simulink model "gif_model"  (R2013a)
settings: Solver=VariableStepDiscrete  StartTime=0.0  StopTime=t_f  RelTol=1e-3
values from neighbouring files (symbols this model uses):
  dt = 1    [test.m]
undefined symbols (not defined in the file or in its folder): filename_main, filename_target, initial_epoch, VERBOSE
libraries: commutil2 x2, dspswit3 x1
settings Model: Creator=Nathan  LastModifiedBy=Adam
settings DataIOCC: LimitDataPoints=off

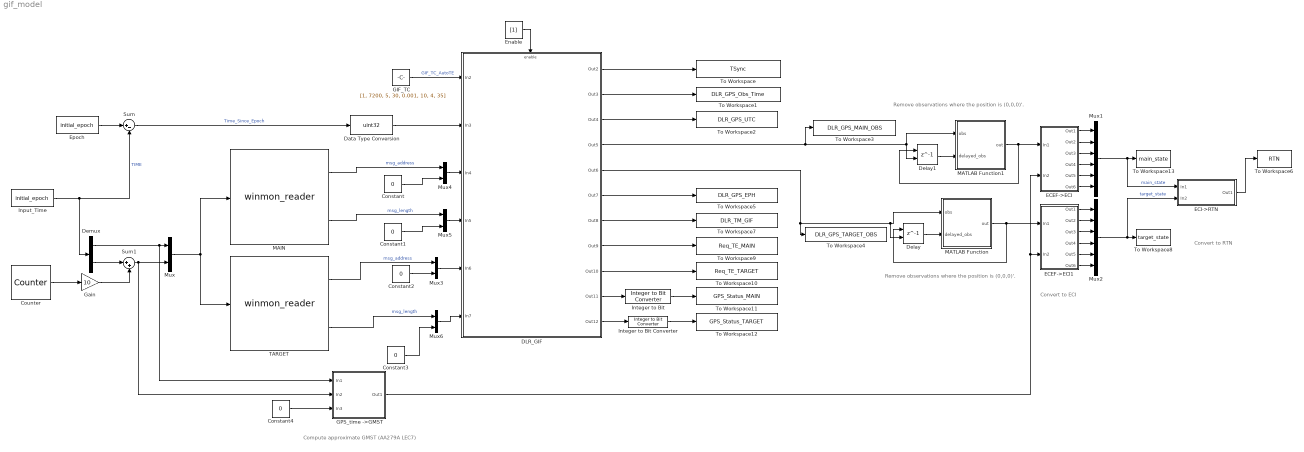
== system gif_model ==
  note: Remove observations where the position is (0,0,0)'.
  note: Convert to RTN
  note: Convert to ECI
  note: Compute approximate GMST
      | (AA279A LEC7)
  note: Remove observations where the position is (0,0,0)'.
  Constant{,1..3} (4 alike) : Constant  Value=0  OutDataTypeStr=uint32
  Constant4 : Constant  Value=0
  Counter : dspswit3/Counter  Direction=Up  CountEvent=Free running  CounterSize=User defined  MaxCount=t_f  InitialCount=0  Output=Count  HitValue=32  ResetInput=off  SamplesPerFrame=1  Ts=10  CntDtype=double  HitDtype=Logical
  DLR_GIF : Subsystem
      mask Display:
      | port_label('input',1,'TC_DLR_GIF')
      | port_label('input',2,'GPS_TIME')
      | port_label('input',3,'GPS_msg_adr_MAIN')
      | port_label('input',4,'GPS_msg_len_MAIN')
      | port_label('input',5,'GPS_msg_adr_TARGET')
      | port_label('input',6,'GPS_msg_len_TARGET')
      | 
      | port_label('output',1,'TSync')
      | port_label('output',2,'DLR_GPS_Obs_Time')
      | port_label('output',3,'DLR_GPS_UTC')
      | port_label('output',4,'DLR_GPS_MAIN_OBS')
      | port_label('output',5,'DLR_GPS_TARGET_OBS')
      | port_label('output',6,'DLR_GPS_EPH')
      | port_label('output',7,'DLR_TM_GIF')
      | port_label('output',8,'Req TE_MAIN')
      | port_label('output',9,'Req TE_TARGET')
      | port_label('output',10,'GPS_Status_MAIN')
      | port_label('output',11,'GPS_Status_TARGET')
  Data Type Conversion : DataTypeConversion  OutDataTypeStr=uint32
  Delay : Delay  DelayLength=1  InitialConditionSource=Input port
      settings: InputPortMap=u0,p4
  Delay1 : Delay  DelayLength=1  InitialConditionSource=Input port
      settings: InputPortMap=u0,p4
  Demux : Demux  Outputs=2
  ECEF->ECI : Subsystem
  ECEF->ECI1 : Subsystem
  ECI->RTN : Subsystem
  Enable : Constant  Value=[1]  OutDataTypeStr=double
  Epoch : Constant  Value=initial_epoch  OutDataTypeStr=double
  "GIF_TC " : Constant  Value=[1, 7200, 5, 30, 0.001, 10, 4, 35]  OutDataTypeStr=double
  GPS_time ->GMST : Subsystem
  Gain : Gain  Gain=10
  "Input_Time " : Constant  Value=initial_epoch  OutDataTypeStr=double
  Integer to Bit : commutil2/Integer to Bit Converter  nbits=7  signedInputValues=Unsigned  bitOrder=MSB first  outDtype=Inherit via internal rule
  Integer to Bit Converter : commutil2/Integer to Bit Converter  nbits=7  signedInputValues=Unsigned  bitOrder=MSB first  outDtype=Inherit via internal rule
  "MAIN " : S-Function  FunctionName=winmon_reader  Parameters=filename_main,dt,VERBOSE  EnableBusSupport=off
  MATLAB Function : MATLAB Function  TreatAsAtomicUnit=on
  MATLAB Function1 : MATLAB Function  TreatAsAtomicUnit=on
  Mux{,3..6} (5 alike) : Mux  Inputs=2
  Mux1 : Mux  Inputs=6
  Mux2 : Mux  Inputs=6
  Sum : Sum  Inputs=|+-
  Sum1 : Sum  Inputs=|++
  TARGET : S-Function  FunctionName=winmon_reader  Parameters=filename_target,dt,VERBOSE  EnableBusSupport=off
  To Workspace : ToWorkspace  VariableName=TSync  SampleTime=-1
  To Workspace1 : ToWorkspace  VariableName=DLR_GPS_Obs_Time  SampleTime=-1
  To Workspace10 : ToWorkspace  VariableName=Req_TE_TARGET  SampleTime=-1
  To Workspace11 : ToWorkspace  VariableName=GPS_Status_MAIN  SampleTime=-1
  To Workspace12 : ToWorkspace  VariableName=GPS_Status_TARGET  SampleTime=-1
  To Workspace13 : ToWorkspace  VariableName=main_state  SampleTime=-1
  To Workspace2 : ToWorkspace  VariableName=DLR_GPS_UTC  SampleTime=-1
  To Workspace3 : ToWorkspace  VariableName=DLR_GPS_MAIN_OBS  SampleTime=-1
  To Workspace4 : ToWorkspace  VariableName=DLR_GPS_TARGET_OBS  SampleTime=-1
  To Workspace5 : ToWorkspace  VariableName=DLR_GPS_EPH  SampleTime=-1
  To Workspace6 : ToWorkspace  VariableName=RTN  SampleTime=-1
  To Workspace7 : ToWorkspace  VariableName=DLR_TM_GIF  SampleTime=-1
  To Workspace8 : ToWorkspace  VariableName=target_state  SampleTime=-1
  To Workspace9 : ToWorkspace  VariableName=Req_TE_MAIN  SampleTime=-1
  wires:
  "Input_Time "/1 -> Demux/1, Sum/2  "TIME"
  Epoch/1 -> Sum/1
  Sum/1 -> Data Type Conversion/1  "Time_Since_Epoch"
  "GIF_TC "/1 -> DLR_GIF/1(In2)  "GIF_TC_AutoTE"
  Enable/1 -> DLR_GIF/Enable
  "MAIN "/1 -> Mux4/1  "msg_address"
  Counter/1 -> Gain/1
  Gain/1 -> Sum1/2
  Demux/2 -> Sum1/1
  Demux/1 -> GPS_time ->GMST/1(In1), Mux/1
  Mux/1 -> "MAIN "/1, TARGET/1
  DLR_GIF/7(Out8) -> To Workspace7/1
  Constant/1 -> Mux4/2
  "MAIN "/2 -> Mux5/1  "msg_length"
  Constant1/1 -> Mux5/2
  TARGET/1 -> Mux3/1  "msg_address"
  Constant2/1 -> Mux3/2
  TARGET/2 -> Mux6/1  "msg_length"
  Constant3/1 -> Mux6/2
  Data Type Conversion/1 -> DLR_GIF/2(In3)
  DLR_GIF/1(Out2) -> To Workspace/1
  DLR_GIF/2(Out3) -> To Workspace1/1
  DLR_GIF/3(Out4) -> To Workspace2/1
  DLR_GIF/4(Out5) -> Delay1/2, MATLAB Function1/1(obs), To Workspace3/1
  DLR_GIF/5(Out6) -> Delay/2, MATLAB Function/1(obs), To Workspace4/1
  DLR_GIF/6(Out7) -> To Workspace5/1
  DLR_GIF/8(Out9) -> To Workspace9/1
  DLR_GIF/9(Out10) -> To Workspace10/1
  ECEF->ECI/1(Out1) -> Mux1/1
  ECEF->ECI/6(Out6) -> Mux1/6
  ECEF->ECI/4(Out4) -> Mux1/4
  ECEF->ECI/3(Out3) -> Mux1/3
  ECEF->ECI/2(Out2) -> Mux1/2
  ECEF->ECI/5(Out5) -> Mux1/5
  Mux1/1 -> ECI->RTN/1(In1), To Workspace13/1  "main_state"
  Sum1/1 -> GPS_time ->GMST/2(In2), Mux/2
  Mux2/1 -> ECI->RTN/2(In2), To Workspace8/1  "target_state"
  ECEF->ECI1/1(Out1) -> Mux2/1
  ECEF->ECI1/3(Out3) -> Mux2/3
  ECEF->ECI1/4(Out4) -> Mux2/4
  ECEF->ECI1/5(Out5) -> Mux2/5
  ECEF->ECI1/2(Out2) -> Mux2/2
  ECEF->ECI1/6(Out6) -> Mux2/6
  Mux6/1 -> DLR_GIF/6(In7)
  Mux4/1 -> DLR_GIF/3(In4)
  Mux5/1 -> DLR_GIF/4(In5)
  Mux3/1 -> DLR_GIF/5(In6)
  ECI->RTN/1(Out1) -> To Workspace6/1
  DLR_GIF/10(Out11) -> Integer to Bit/1
  Integer to Bit/1 -> To Workspace11/1
  DLR_GIF/11(Out12) -> Integer to Bit Converter/1
  Integer to Bit Converter/1 -> To Workspace12/1
  Delay/1 -> MATLAB Function/2(delayed_obs)
  MATLAB Function/1(out) -> Delay/1, ECEF->ECI1/1(In1)
  MATLAB Function1/1(out) -> Delay1/1, ECEF->ECI/1(In1)
  Delay1/1 -> MATLAB Function1/2(delayed_obs)
  GPS_time ->GMST/1(Out1) -> ECEF->ECI/2(In2), ECEF->ECI1/2(In2)
  Constant4/1 -> GPS_time ->GMST/3(In3)

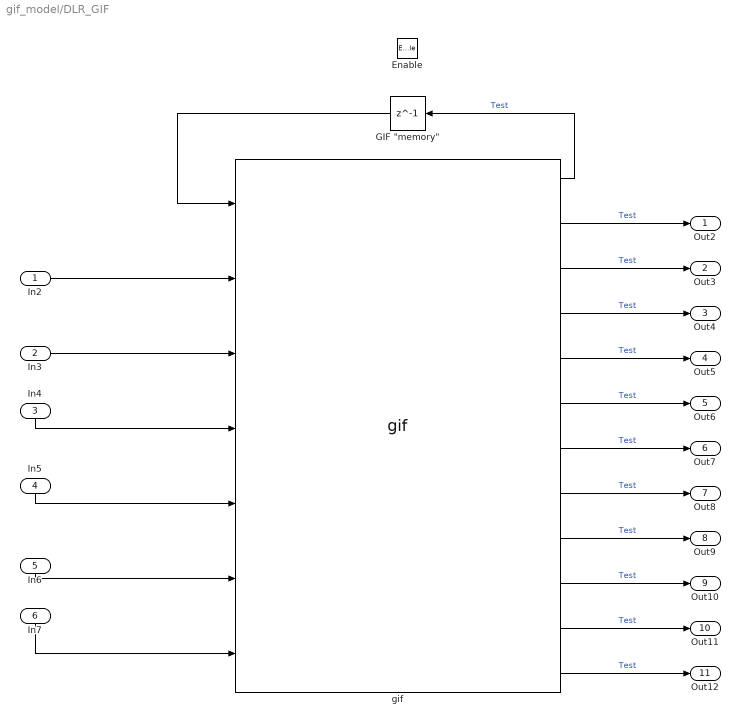
== system gif_model/DLR_GIF ==
  In2 : Inport
  In3 : Inport  Port=2
  In4 : Inport  Port=3
  In5 : Inport  Port=4
  In6 : Inport  Port=5
  In7 : Inport  Port=6
  Enable : EnablePort  StatesWhenEnabling=reset
  "GIF \"memory\"" : Delay  DelayLength=1  InitialCondition=0
  gif : S-Function  FunctionName=gif  EnableBusSupport=off
      mask Display:
      | port_label('input',1,'MEM_in')
      | port_label('input',2,'TC_DLR_GIF')
      | port_label('input',3,'GPS_TIME')
      | port_label('input',4,'GPS_msg_adr_MAIN')
      | port_label('input',5,'GPS_msg_len_MAIN')
      | port_label('input',6,'GPS_msg_adr_TARGET')
      | port_label('input',7,'GPS_msg_len_TARGET')
      | 
      | port_label('output',1,'MEM_out')
      | port_label('output',2,'TSync')
      | port_label('output',3,'DLR_GPS_Obs_Time')
      | port_label('output',4,'DLR_GPS_UTC')
      | port_label('output',5,'DLR_GPS_MAIN_OBS')
      | port_label('output',6,'DLR_GPS_TARGET_OBS')
      | port_label('output',7,'DLR_GPS_EPH')
      | port_label('output',8,'DLR_TM_GIF')
      | port_label('output',9,'Req TE_MAIN')
      | port_label('output',10,'Req TE_TARGET')
      | port_label('output',11,'GPS_Status_MAIN')
      | port_label('output',12,'GPS_Status_TARGET')
  Out2 : Outport
  Out3 : Outport  Port=2
  Out4 : Outport  Port=3
  Out5 : Outport  Port=4
  Out6 : Outport  Port=5
  Out7 : Outport  Port=6
  Out8 : Outport  Port=7
  Out9 : Outport  Port=8
  Out10 : Outport  Port=9
  Out11 : Outport  Port=10
  Out12 : Outport  Port=11
  wires:
  In5/1 -> gif/5
  In4/1 -> gif/4
  In7/1 -> gif/7
  In6/1 -> gif/6
  In2/1 -> gif/2
  gif/5 -> Out5/1  "Test"
  gif/6 -> Out6/1  "Test"
  gif/7 -> Out7/1  "Test"
  gif/3 -> Out3/1  "Test"
  gif/4 -> Out4/1  "Test"
  gif/12 -> Out12/1  "Test"
  gif/2 -> Out2/1  "Test"
  gif/10 -> Out10/1  "Test"
  gif/11 -> Out11/1  "Test"
  gif/8 -> Out8/1  "Test"
  gif/9 -> Out9/1  "Test"
  In3/1 -> gif/3
  gif/1 -> "GIF \"memory\""/1  "Test"
  "GIF \"memory\""/1 -> gif/1

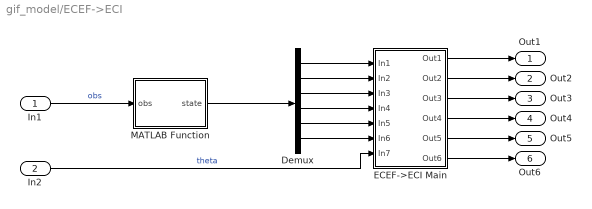
== system gif_model/ECEF->ECI ==
  In1 : Inport
  In2 : Inport  Port=2
  Demux : Demux  Outputs=6
  ECEF->ECI Main : Subsystem
  MATLAB Function : MATLAB Function  TreatAsAtomicUnit=on
  Out1 : Outport
  Out2 : Outport  Port=2
  Out3 : Outport  Port=3
  Out4 : Outport  Port=4
  Out5 : Outport  Port=5
  Out6 : Outport  Port=6
  wires:
  ECEF->ECI Main/1(Out1) -> Out1/1
  ECEF->ECI Main/2(Out2) -> Out2/1
  ECEF->ECI Main/3(Out3) -> Out3/1
  ECEF->ECI Main/4(Out4) -> Out4/1
  ECEF->ECI Main/5(Out5) -> Out5/1
  ECEF->ECI Main/6(Out6) -> Out6/1
  In1/1 -> MATLAB Function/1(obs)  "obs"
  In2/1 -> ECEF->ECI Main/7(In7)  "theta"
  MATLAB Function/1(state) -> Demux/1
  Demux/6 -> ECEF->ECI Main/6(In6)
  Demux/3 -> ECEF->ECI Main/3(In3)
  Demux/4 -> ECEF->ECI Main/4(In4)
  Demux/5 -> ECEF->ECI Main/5(In5)
  Demux/2 -> ECEF->ECI Main/2(In2)
  Demux/1 -> ECEF->ECI Main/1(In1)

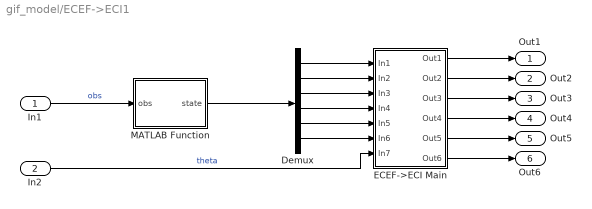
== system gif_model/ECEF->ECI1 ==
  In1 : Inport
  In2 : Inport  Port=2
  Demux : Demux  Outputs=6
  ECEF->ECI Main : Subsystem
  MATLAB Function : MATLAB Function  TreatAsAtomicUnit=on
  Out1 : Outport
  Out2 : Outport  Port=2
  Out3 : Outport  Port=3
  Out4 : Outport  Port=4
  Out5 : Outport  Port=5
  Out6 : Outport  Port=6
  wires:
  ECEF->ECI Main/1(Out1) -> Out1/1
  ECEF->ECI Main/2(Out2) -> Out2/1
  ECEF->ECI Main/3(Out3) -> Out3/1
  ECEF->ECI Main/4(Out4) -> Out4/1
  ECEF->ECI Main/5(Out5) -> Out5/1
  ECEF->ECI Main/6(Out6) -> Out6/1
  In1/1 -> MATLAB Function/1(obs)  "obs"
  In2/1 -> ECEF->ECI Main/7(In7)  "theta"
  MATLAB Function/1(state) -> Demux/1
  Demux/6 -> ECEF->ECI Main/6(In6)
  Demux/3 -> ECEF->ECI Main/3(In3)
  Demux/4 -> ECEF->ECI Main/4(In4)
  Demux/5 -> ECEF->ECI Main/5(In5)
  Demux/2 -> ECEF->ECI Main/2(In2)
  Demux/1 -> ECEF->ECI Main/1(In1)

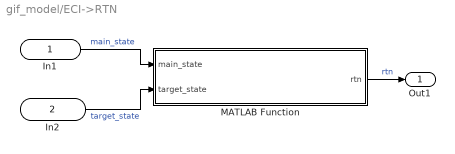
== system gif_model/ECI->RTN ==
  In1 : Inport
  In2 : Inport  Port=2
  MATLAB Function : MATLAB Function  TreatAsAtomicUnit=on
  Out1 : Outport
  wires:
  MATLAB Function/1(rtn) -> Out1/1  "rtn"
  In1/1 -> MATLAB Function/1(main_state)  "main_state"
  In2/1 -> MATLAB Function/2(target_state)  "target_state"

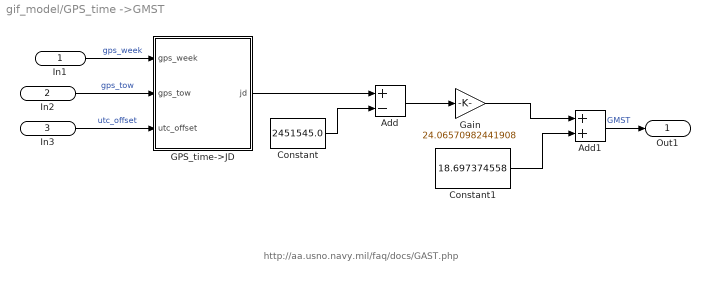
== system gif_model/GPS_time ->GMST ==
  note: http://aa.usno.navy.mil/faq/docs/GAST.php
  In1 : Inport
  In2 : Inport  Port=2
  In3 : Inport  Port=3
  " GPS_time->JD" : MATLAB Function  TreatAsAtomicUnit=on
  Add : Sum  Inputs=+-
  Add1 : Sum
  Constant : Constant  Value=2451545.0
  Constant1 : Constant  Value=18.697374558
  Gain : Gain  Gain=24.06570982441908
  Out1 : Outport
  wires:
  In2/1 -> " GPS_time->JD"/2(gps_tow)  "gps_tow"
  In1/1 -> " GPS_time->JD"/1(gps_week)  "gps_week"
  " GPS_time->JD"/1(jd) -> Add/1
  Constant/1 -> Add/2
  Add/1 -> Gain/1
  Gain/1 -> Add1/1
  Constant1/1 -> Add1/2
  Add1/1 -> Out1/1  "GMST"
  In3/1 -> " GPS_time->JD"/3(utc_offset)  "utc_offset"

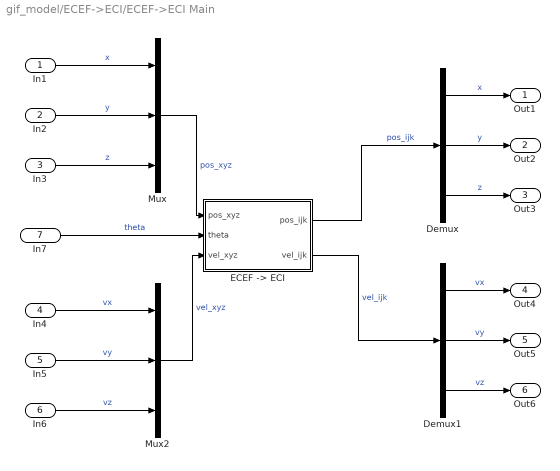
== system gif_model/ECEF->ECI/ECEF->ECI Main ==
  In1 : Inport
  In2 : Inport  Port=2
  In3 : Inport  Port=3
  In4 : Inport  Port=4
  In5 : Inport  Port=5
  In6 : Inport  Port=6
  In7 : Inport  Port=7
  Demux : Demux  Outputs=3
  Demux1 : Demux  Outputs=3
  "ECEF -> ECI" : MATLAB Function  TreatAsAtomicUnit=on
  Mux : Mux  Inputs=3
  Mux2 : Mux  Inputs=3
  Out1 : Outport
  Out2 : Outport  Port=2
  Out3 : Outport  Port=3
  Out4 : Outport  Port=4
  Out5 : Outport  Port=5
  Out6 : Outport  Port=6
  wires:
  In3/1 -> Mux/3  "z"
  In6/1 -> Mux2/3  "vz"
  In4/1 -> Mux2/1  "vx"
  In2/1 -> Mux/2  "y"
  In5/1 -> Mux2/2  "vy"
  In1/1 -> Mux/1  "x"
  In7/1 -> "ECEF -> ECI"/2(theta)  "theta"
  "ECEF -> ECI"/2(vel_ijk) -> Demux1/1  "vel_ijk"
  Demux1/1 -> Out4/1  "vx"
  Demux1/2 -> Out5/1  "vy"
  Demux/1 -> Out1/1  "x"
  Demux/2 -> Out2/1  "y"
  Demux/3 -> Out3/1  "z"
  "ECEF -> ECI"/1(pos_ijk) -> Demux/1  "pos_ijk"
  Mux/1 -> "ECEF -> ECI"/1(pos_xyz)  "pos_xyz"
  Mux2/1 -> "ECEF -> ECI"/3(vel_xyz)  "vel_xyz"
  Demux1/3 -> Out6/1  "vz"

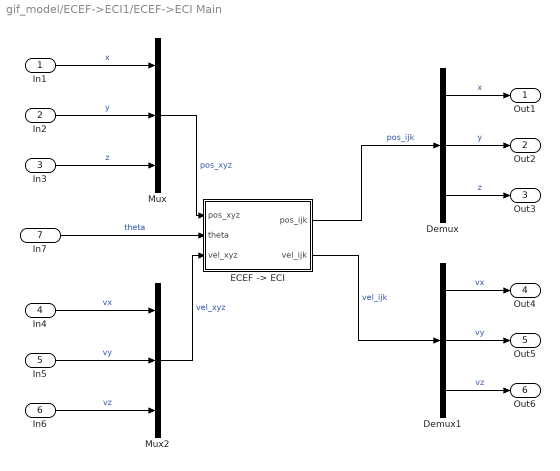
== system gif_model/ECEF->ECI1/ECEF->ECI Main ==
  In1 : Inport
  In2 : Inport  Port=2
  In3 : Inport  Port=3
  In4 : Inport  Port=4
  In5 : Inport  Port=5
  In6 : Inport  Port=6
  In7 : Inport  Port=7
  Demux : Demux  Outputs=3
  Demux1 : Demux  Outputs=3
  "ECEF -> ECI" : MATLAB Function  TreatAsAtomicUnit=on
  Mux : Mux  Inputs=3
  Mux2 : Mux  Inputs=3
  Out1 : Outport
  Out2 : Outport  Port=2
  Out3 : Outport  Port=3
  Out4 : Outport  Port=4
  Out5 : Outport  Port=5
  Out6 : Outport  Port=6
  wires:
  In3/1 -> Mux/3  "z"
  In6/1 -> Mux2/3  "vz"
  In4/1 -> Mux2/1  "vx"
  In2/1 -> Mux/2  "y"
  In5/1 -> Mux2/2  "vy"
  In1/1 -> Mux/1  "x"
  In7/1 -> "ECEF -> ECI"/2(theta)  "theta"
  "ECEF -> ECI"/2(vel_ijk) -> Demux1/1  "vel_ijk"
  Demux1/1 -> Out4/1  "vx"
  Demux1/2 -> Out5/1  "vy"
  Demux/1 -> Out1/1  "x"
  Demux/2 -> Out2/1  "y"
  Demux/3 -> Out3/1  "z"
  "ECEF -> ECI"/1(pos_ijk) -> Demux/1  "pos_ijk"
  Mux/1 -> "ECEF -> ECI"/1(pos_xyz)  "pos_xyz"
  Mux2/1 -> "ECEF -> ECI"/3(vel_xyz)  "vel_xyz"
  Demux1/3 -> Out6/1  "vz"

== matlab function gif_model/ECEF->ECI/ECEF->ECI Main/ECEF -> ECI ==
  data: pos_xyz input; theta input; pos_ijk output; vel_xyz input; vel_ijk output
function [pos_ijk, vel_ijk] = fcn(pos_xyz,theta,vel_xyz)
%Convert position and velocity in ECEF(_xyz) to ECI(_ijk)

%Rotation matrix
R = [cos(theta), sin(theta), 0;
     -sin(theta), cos(theta),0;
     0, 0, 1];
rot_xyz_to_ijk = R';
pos_ijk = rot_xyz_to_ijk*pos_xyz;

w = [0;0;theta];
vel_ijk = rot_xyz_to_ijk*(vel_xyz + cross(w,pos_xyz));
end

== matlab function gif_model/GPS_time ->GMST/ GPS_time->JD ==
  data: gps_week input; jd output; gps_tow input; utc_offset input
function jd  = gps_to_jd(gps_week,gps_tow, utc_offset)
%convert GPS week and seconds of the week to Julian Date
%gps_week,      //!< GPS week (0-1024+)             [week]
%gps_tow,       //!< GPS time of week (0-604800.0)  [s]
%utc_offset,    //!< Integer seconds that GPS is ahead of UTC time, always positive [s]
%julian_date    //!< Number of days since noon Universal Time Jan 1, 4713 BCE (Julian calendar) [days]

JULIAN_DATE_START_OF_GPS_TIME = 2444244.5;

jd = (gps_week + (gps_tow-utc_offset)/604800.0)*7.0 + ...
    JULIAN_DATE_START_OF_GPS_TIME;
end

== matlab function gif_model/ECEF->ECI/MATLAB Function ==
  data: obs input; state output
function state = fcn(obs)
%Select the position and velocity observables

state = obs(16:21);
end

== matlab function gif_model/ECEF->ECI1/ECEF->ECI Main/ECEF -> ECI ==
  data: pos_xyz input; theta input; pos_ijk output; vel_xyz input; vel_ijk output
function [pos_ijk, vel_ijk] = fcn(pos_xyz,theta,vel_xyz)
%Convert position and velocity in ECEF(_xyz) to ECI(_ijk)

%Rotation matrix
R = [cos(theta), sin(theta), 0;
     -sin(theta), cos(theta),0;
     0, 0, 1];
rot_xyz_to_ijk = R';
pos_ijk = rot_xyz_to_ijk*pos_xyz;

w = [0;0;theta];
vel_ijk = rot_xyz_to_ijk*(vel_xyz + cross(w,pos_xyz));
end

== matlab function gif_model/ECEF->ECI1/MATLAB Function ==
  data: obs input; state output
function state = fcn(obs)
%Select the position and velocity observables

state = obs(16:21);
end

== matlab function gif_model/ECI->RTN/MATLAB Function ==
  data: main_state input; rtn output; target_state input
function rtn = compute_rtn(main_state,target_state)
%convert positions of Main and Target in ECI to relative position in RTN

%extract required data to easily manageable form
main = struct('pos_RTN',zeros(3,1),'pos',zeros(3,1),'vel',zeros(3,1));
trgt = struct('pos_RTN',zeros(3,1),'pos',zeros(3,1),'vel',zeros(3,1));

main.pos = main_state(1:3);
main.vel = main_state(4:6);
trgt.pos = target_state(1:3);
trgt.vel = target_state(4:6);

%compute rotation matrix
R_IJK = (main.pos/norm(main.pos));
N_IJK = (cross(main.pos,main.vel)/norm(cross(main.pos,main.vel)));
T_IJK = (cross(N_IJK,R_IJK));

rot_RTN_to_IJK = [R_IJK,T_IJK,N_IJK];
rot_IJK_to_RTN = rot_RTN_to_IJK';

%angular velocity of RTN wrt IJK should be normal to chief's orbital plane
%TODO: angular velocity of RTN wrt IJK

%rotate both positions to RTN frame and subtract
main.pos_RTN = rot_IJK_to_RTN*main.pos;
trgt.pos_RTN = rot_IJK_to_RTN*trgt.pos;
rtn = trgt.pos_RTN-main.pos_RTN;

end

== matlab function gif_model/MATLAB Function ==
  data: obs input; out output; delayed_obs input
function out = delay_switcher(obs, delayed_obs)
%Remove states with a position fix of [0;0;0]

if min(obs(16:18)==[0,0,0]')==1
    out = delayed_obs;
else
    out = obs;
end
end

== matlab function gif_model/MATLAB Function1 ==
  data: obs input; out output; delayed_obs input
function out = delay_switcher(obs, delayed_obs)
%Remove states with a position of [0;0;0]

if min(obs(16:18)==[0,0,0]')==1
    out = delayed_obs;
else
    out = obs;
end
end
